simulink model "Workshop1"  (R2021a)
settings: Solver=VariableStepAuto  StartTime=0.0  StopTime=10.0  RelTol=1e-3
libraries: simulink x1
settings Model: SnapshotBufferSize=1  SnapshotInterval=1  Creator=ZYT  LastModifiedBy=ZYT

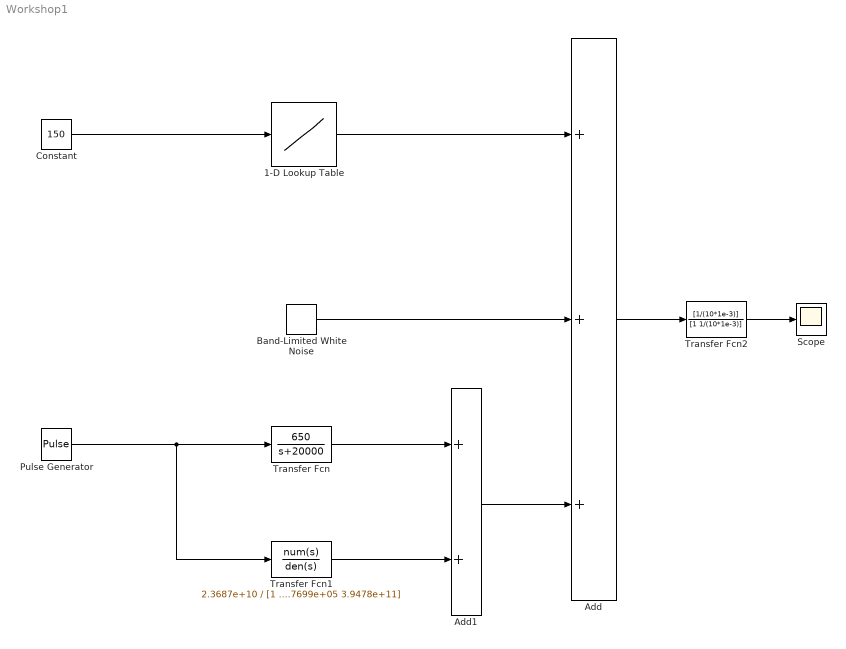
== system Workshop1 ==
  1-D Lookup Table : Lookup_n-D  NumberOfTableDimensions=1  BreakpointsForDimension1=[20 150]  Table=[2.45 0.4]  InternalRulePriority=Speed  RndMeth=Simplest  InputSameDT=on
  Add : Sum  Inputs=+++
  Add1 : Sum
  Band-Limited White Noise : simulink/Sources/Band-Limited White Noise  Cov=[0.0000000001]  Ts=8.0000e-07  seed=[23341]
  Constant : Constant  Value=150
  Pulse Generator : DiscretePulseGenerator  PulseType=Time based  Amplitude=0.1  Period=0.001  PulseWidth=13
  Scope : Scope
  Transfer Fcn : TransferFcn  Numerator=[650]  Denominator=[1 20000]
  Transfer Fcn1 : TransferFcn  Numerator=2.3687e+10  Denominator=[1 3.7699e+05 3.9478e+11]
  Transfer Fcn2 : TransferFcn  Numerator=[1/(10*1e-3)]  Denominator=[1 1/(10*1e-3)]
  wires:
  Pulse Generator/1 -> Transfer Fcn/1, Transfer Fcn1/1
  Constant/1 -> 1-D Lookup Table/1
  1-D Lookup Table/1 -> Add/1
  Band-Limited White Noise/1 -> Add/2
  Transfer Fcn/1 -> Add1/1
  Transfer Fcn1/1 -> Add1/2
  Add1/1 -> Add/3
  Add/1 -> Transfer Fcn2/1
  Transfer Fcn2/1 -> Scope/1
